simulink model "carrier_frequency"  (R2021a)
settings: Solver=VariableStepAuto  StartTime=0.0  StopTime=20/fsw  MaxStep=1e-7  RelTol=1e-6
InitFcn:
  | fsw=10e3;
  | ma=0.50;
  | ffund=100;
libraries: spsFourierLib x1
settings Model: Creator=enes_  LastModifiedBy=enes_
settings DataIOCC: SaveFormat=StructureWithTime  ReturnWorkspaceOutputs=off

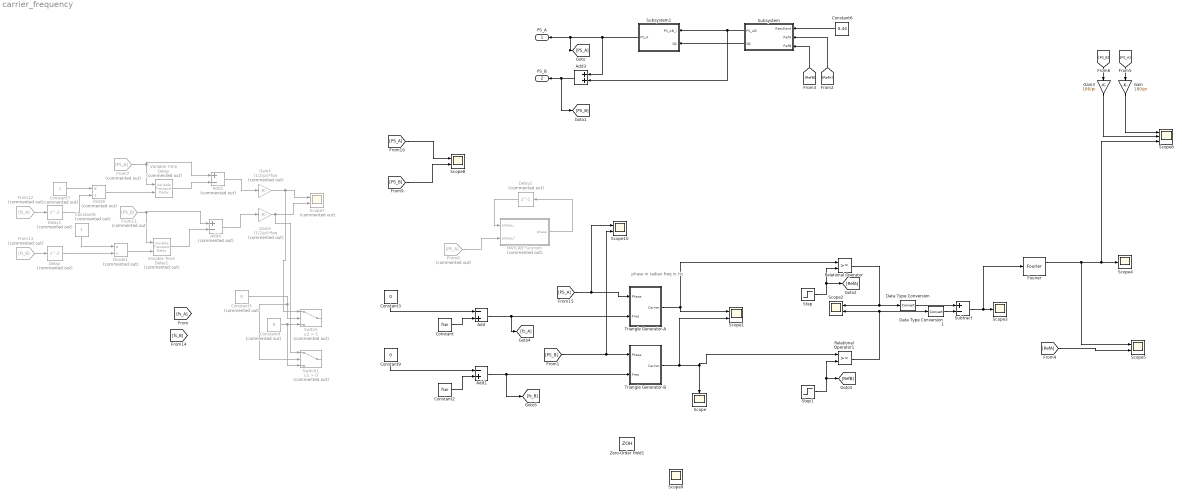
== system carrier_frequency ==
  note: phase in radian
      | freq in Hz
  Add : Sum  Inputs=-+
  Add1 : Sum  Inputs=-+
  Add2 : Sum  Commented=on  Inputs=+-
  Add3 : Sum
  Add4 : Sum  Commented=on  Inputs=+-
  Constant : Constant  Value=fsw
  Constant2 : Constant  Value=fsw
  Constant3 : Constant  Value=0
  Constant4 : Constant  Commented=on  Value=0
  Constant5 : Constant  Commented=on  Value=0
  Constant6 : Constant  Value=0.44
  Constant7 : Constant  Commented=on
  Constant8 : Constant  Commented=on
  Constant9 : Constant  Value=0
  Data Type Conversion : DataTypeConversion
  Data Type Conversion1 : DataTypeConversion
  Delay : Delay  Commented=on
  Delay1 : Delay  Commented=on
  Delay2 : Delay  Commented=on  DelayLength=1
  Divide : Product  Commented=on  Inputs=*/
  Divide1 : Product  Commented=on  Inputs=*/
  Fourier : spsFourierLib/Fourier  Freq=fsw  n=1  InInit=[0, 0]  Ts=0
      settings: SourceProductBaseCode=PS
  From11 : From  Commented=on  GotoTag=PS_B
  From12 : From  Commented=on  GotoTag=fs_A
  From13 : From  Commented=on  GotoTag=fs_B
  From7 : From  Commented=on  GotoTag=PS_A
  From8 : From  Commented=on  GotoTag=PS_A
  Gain : Gain  Gain=180/pi
  Gain3 : Gain  Gain=180/pi
  Gain4 : Gain  Commented=on  Gain=(1/2/pi)*fsw
  Gain5 : Gain  Commented=on  Gain=(1/2/pi)*fsw
  MATLAB Function : MATLAB Function  Commented=on  TreatAsAtomicUnit=on
  Relational Operator : RelationalOperator  OutDataTypeStr=boolean  RndMeth=Simplest
  Relational Operator1 : RelationalOperator  OutDataTypeStr=boolean  RndMeth=Simplest
  Scope : Scope
  Scope{1..2,5,8..10} (6 alike) : Scope  NumInputPorts=2
  Scope3 : Scope
  Scope4 : Scope
  Scope6 : Scope  NumInputPorts=3
  Scope7 : Scope  Commented=on  NumInputPorts=2
  Step : Step  Time=5/fsw  Before=0.5  After=0.25  SampleTime=0
  Step1 : Step  Time=5/fsw  Before=0.25  After=0.5  SampleTime=0
  Subsystem : Subsystem
  Subsystem1 : Subsystem
  Subtract : Sum  Inputs=+-
  Switch : Switch  Commented=on  Criteria=u2 > Threshold  Threshold=5
  Switch1 : Switch  Commented=on  Criteria=u2 > Threshold
  Triangle Generator-A : Subsystem
  Triangle Generator-B : Subsystem
  Variable Time Delay : VariableTransportDelay  Commented=on  MaximumDelay=10
  Variable Time Delay1 : VariableTransportDelay  Commented=on  MaximumDelay=10
  Zero-Order Hold1 : ZeroOrderHold  SampleTime=1/fsw
  PS_A : Outport
  PS_B : Outport  Port=2
  wires:
  Add1/1 -> [fs_B], Triangle Generator-B/2(Freq)
  Step/1 -> [RefA], Relational Operator/2
  Triangle Generator-B/1(Carrier) -> Scope1/2, Scope/1, Relational Operator1/1
  Triangle Generator-A/1(Carrier) -> Scope1/1, Relational Operator/1
  Step1/1 -> Relational Operator1/2, [RefB]
  Add/1 -> [fs_A], Triangle Generator-A/2(Freq)
  Constant/1 -> Add/2
  Gain4/1 -> Switch/1, Scope7/1
  Gain5/1 -> Switch1/1, Scope7/2
  Constant2/1 -> Add1/2
  Relational Operator/1 -> Data Type Conversion/1, Scope2/1
  Relational Operator1/1 -> Scope2/2, Data Type Conversion1/1
  Subtract/1 -> Fourier/1, Scope3/1
  Data Type Conversion/1 -> Subtract/1
  Data Type Conversion1/1 -> Subtract/2
  Fourier/1 -> Scope5/1, Scope6/3, Scope4/1
  Constant6/1 -> Subsystem/1(Resultant)
  Subsystem/1(PS_AB) -> Add3/2, Subsystem1/1(PS_AB_i)
  Subsystem/2(SB) -> Subsystem1/2(SB)
  Subsystem1/1(PS_A) -> Add3/1, [PS_A], PS_A/1
  Add3/1 -> [PS_B], PS_B/1
  [RefA] -> Subsystem/2(RefA)
  [RefB] -> Subsystem/3(RefB)
  [RefA] -> Scope5/2
  [PS_A] -> Gain/1
  Gain/1 -> Scope6/1
  Gain3/1 -> Scope6/2
  [PS_B] -> Gain3/1
  Add4/1 -> Gain5/1
  [PS_A] -> Scope8/1
  [PS_B] -> Scope8/2
  Variable Time Delay/1 -> Add2/2
  From7/1 -> Add2/1, Variable Time Delay/1
  Add2/1 -> Gain4/1
  Variable Time Delay1/1 -> Add4/2
  From11/1 -> Add4/1, Variable Time Delay1/1
  Constant4/1 -> Switch1/3, Switch/3
  Constant5/1 -> Switch1/2, Switch/2
  Constant7/1 -> Divide/1
  Divide/1 -> Variable Time Delay/2
  Divide1/1 -> Variable Time Delay1/2
  Constant8/1 -> Divide1/1
  [PS_B] -> Triangle Generator-B/1(Phase), Scope10/2
  From13/1 -> Delay/1
  Delay/1 -> Divide1/2
  From12/1 -> Delay1/1
  Delay1/1 -> Divide/2
  Delay2/1 -> MATLAB Function/1(phase_i)
  From8/1 -> MATLAB Function/2(phase_f)
  MATLAB Function/1(phase) -> Delay2/1
  Constant3/1 -> Add/1
  Constant9/1 -> Add1/1
  [PS_A] -> Scope10/1, Triangle Generator-A/1(Phase)

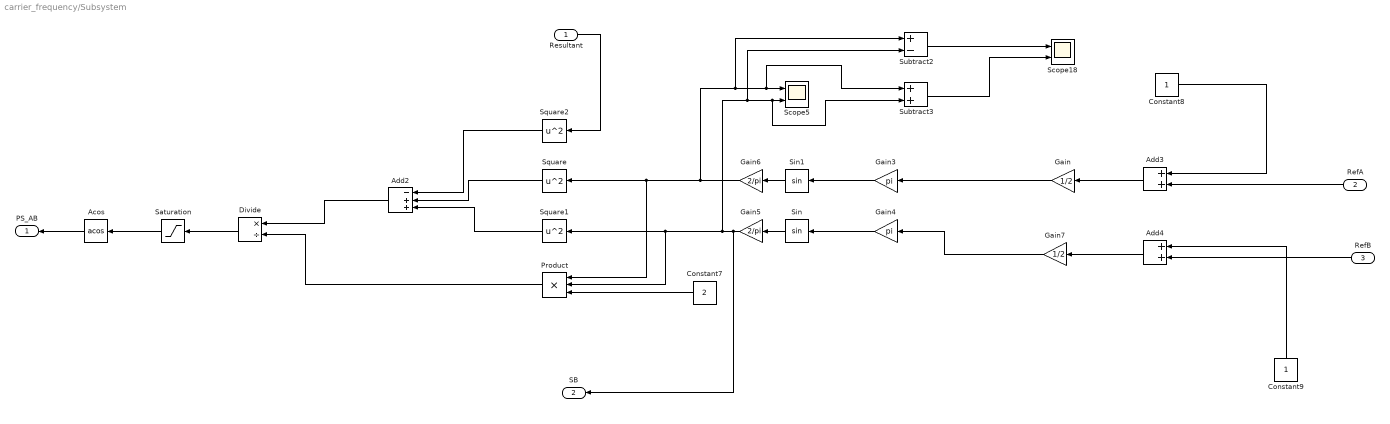
== system carrier_frequency/Subsystem ==
  Resultant : Inport
  RefA : Inport  Port=2
  RefB : Inport  Port=3
  Acos : Trigonometry  Operator=acos
  Add2 : Sum  Inputs=-++
  Add3 : Sum
  Add4 : Sum
  Constant7 : Constant  Value=2
  Constant8 : Constant
  Constant9 : Constant
  Divide : Product  Inputs=*/
  Gain : Gain  Gain=1/2
  Gain3 : Gain  Gain=pi
  Gain4 : Gain  Gain=pi
  Gain5 : Gain  Gain=2/pi
  Gain6 : Gain  Gain=2/pi
  Gain7 : Gain  Gain=1/2
  Product : Product  Inputs=3
  Saturation : Saturate  UpperLimit=1  LowerLimit=-1
  Scope18 : Scope  NumInputPorts=2
  Scope5 : Scope  NumInputPorts=2
  Sin : Trigonometry
  Sin1 : Trigonometry
  Square : Math  Operator=square  SaturateOnIntegerOverflow=on
  Square1 : Math  Operator=square  SaturateOnIntegerOverflow=on
  Square2 : Math  Operator=square  SaturateOnIntegerOverflow=on
  Subtract2 : Sum  Inputs=+-
  Subtract3 : Sum
  PS_AB : Outport
  SB : Outport  Port=2
  wires:
  Acos/1 -> PS_AB/1
  Add3/1 -> Gain/1
  Constant8/1 -> Add3/1
  Gain6/1 -> Subtract2/1, Subtract3/1, Scope5/1, Product/1, Square/1
  Constant9/1 -> Add4/1
  RefA/1 -> Add3/2
  Gain7/1 -> Gain4/1
  Gain5/1 -> Product/2, Square1/1, Subtract2/2, Subtract3/2, Scope5/2, SB/1
  Gain4/1 -> Sin/1
  Add4/1 -> Gain7/1
  Subtract3/1 -> Scope18/2
  Saturation/1 -> Acos/1
  Constant7/1 -> Product/3
  Gain/1 -> Gain3/1
  RefB/1 -> Add4/2
  Add2/1 -> Divide/1
  Resultant/1 -> Square2/1
  Divide/1 -> Saturation/1
  Sin/1 -> Gain5/1
  Sin1/1 -> Gain6/1
  Subtract2/1 -> Scope18/1
  Product/1 -> Divide/2
  Gain3/1 -> Sin1/1
  Square2/1 -> Add2/1
  Square1/1 -> Add2/3
  Square/1 -> Add2/2

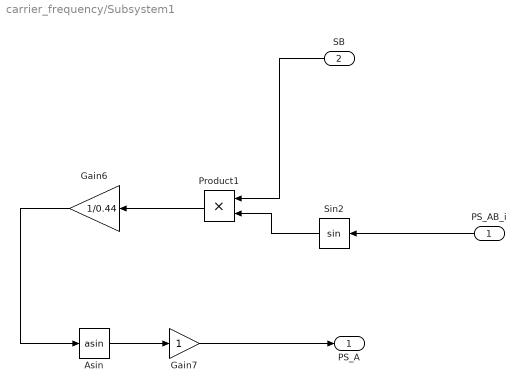
== system carrier_frequency/Subsystem1 ==
  PS_AB_i : Inport
  SB : Inport  Port=2
  Asin : Trigonometry  Operator=asin
  Gain6 : Gain  Gain=1/0.44
  Gain7 : Gain
  Product1 : Product
  Sin2 : Trigonometry
  PS_A : Outport
  wires:
  SB/1 -> Product1/1
  Asin/1 -> Gain7/1
  Gain6/1 -> Asin/1
  Sin2/1 -> Product1/2
  Product1/1 -> Gain6/1
  Gain7/1 -> PS_A/1
  PS_AB_i/1 -> Sin2/1

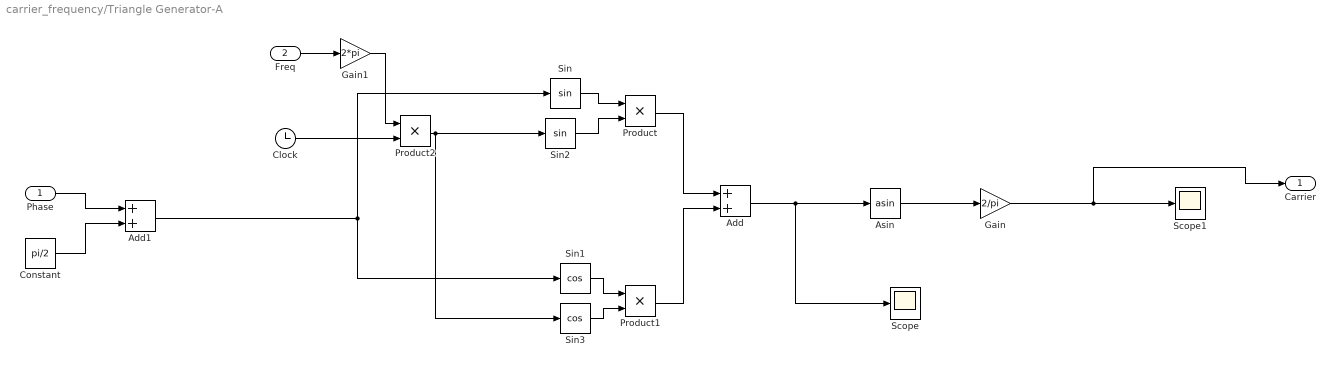
== system carrier_frequency/Triangle Generator-A ==
  Phase : Inport
  Freq : Inport  Port=2
  Add : Sum
  Add1 : Sum
  Asin : Trigonometry  Operator=asin
  Clock : Clock
  Constant : Constant  Value=pi/2
  Gain : Gain  Gain=2/pi
  Gain1 : Gain  Gain=2*pi
  Product : Product
  Product1 : Product
  Product2 : Product
  Scope : Scope
  Scope1 : Scope
  Sin : Trigonometry
  Sin1 : Trigonometry  Operator=cos
  Sin2 : Trigonometry
  Sin3 : Trigonometry  Operator=cos
  Carrier : Outport
  wires:
  Sin/1 -> Product/1
  Sin2/1 -> Product/2
  Product/1 -> Add/1
  Asin/1 -> Gain/1
  Product1/1 -> Add/2
  Add/1 -> Asin/1, Scope/1
  Sin1/1 -> Product1/1
  Freq/1 -> Gain1/1
  Gain1/1 -> Product2/1
  Clock/1 -> Product2/2
  Sin3/1 -> Product1/2
  Product2/1 -> Sin3/1, Sin2/1
  Gain/1 -> Scope1/1, Carrier/1
  Add1/1 -> Sin/1, Sin1/1
  Constant/1 -> Add1/2
  Phase/1 -> Add1/1

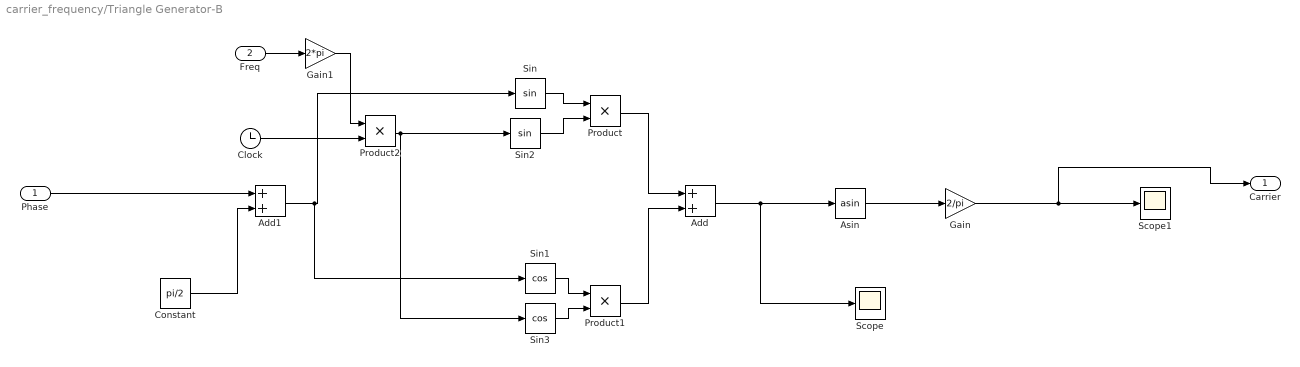
== system carrier_frequency/Triangle Generator-B ==
  Phase : Inport
  Freq : Inport  Port=2
  Add : Sum
  Add1 : Sum
  Asin : Trigonometry  Operator=asin
  Clock : Clock
  Constant : Constant  Value=pi/2
  Gain : Gain  Gain=2/pi
  Gain1 : Gain  Gain=2*pi
  Product : Product
  Product1 : Product
  Product2 : Product
  Scope : Scope
  Scope1 : Scope
  Sin : Trigonometry
  Sin1 : Trigonometry  Operator=cos
  Sin2 : Trigonometry
  Sin3 : Trigonometry  Operator=cos
  Carrier : Outport
  wires:
  Sin/1 -> Product/1
  Sin2/1 -> Product/2
  Product/1 -> Add/1
  Asin/1 -> Gain/1
  Product1/1 -> Add/2
  Add/1 -> Asin/1, Scope/1
  Sin1/1 -> Product1/1
  Freq/1 -> Gain1/1
  Gain1/1 -> Product2/1
  Clock/1 -> Product2/2
  Sin3/1 -> Product1/2
  Product2/1 -> Sin3/1, Sin2/1
  Gain/1 -> Scope1/1, Carrier/1
  Add1/1 -> Sin1/1, Sin/1
  Constant/1 -> Add1/2
  Phase/1 -> Add1/1

== matlab function carrier_frequency/MATLAB Function ==
  data: phase_i input; phase output; phase_f input
function phase  = fcn(phase_i,phase_f)

phase= phase_i + (phase_f-phase_i)/5;
